simulink model "prob4"  (R2020a)
settings: Solver=VariableStepAuto  StartTime=0.0  StopTime=10.0  RelTol=1e-3
settings Model: DataDictionary=data.sldd  Creator=vijay  LastModifiedBy=vijay

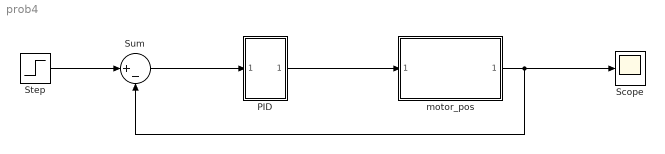
== system prob4 ==
  PID : Subsystem
  Scope : Scope
  Step : Step  Time=0  SampleTime=0
  Sum : Sum  Inputs=|+-
  motor_pos : Subsystem  TreatAsAtomicUnit=on  ReferencedSubsystem=motor_pos
  wires:
  motor_pos/1 -> Sum/2, Scope/1
  Step/1 -> Sum/1
  Sum/1 -> PID/1(In1)
  PID/1(Out1) -> motor_pos/1

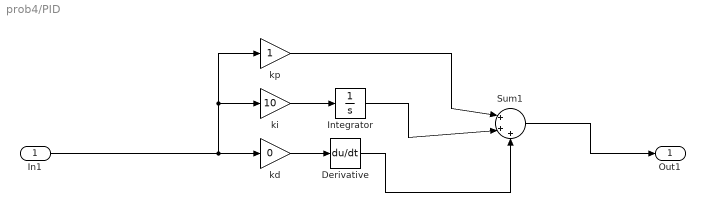
== system prob4/PID ==
  In1 : Inport
  Derivative : Derivative
  Integrator : Integrator
  Sum1 : Sum  Inputs=|+++
  kd : Gain  Gain=0
  ki : Gain  Gain=10
  kp : Gain
  Out1 : Outport
  wires:
  kp/1 -> Sum1/1
  ki/1 -> Integrator/1
  Integrator/1 -> Sum1/2
  kd/1 -> Derivative/1
  Sum1/1 -> Out1/1
  Derivative/1 -> Sum1/3
  In1/1 -> kd/1, ki/1, kp/1
